simulink model "MPCtest3"  (Simulink 7.9)
settings: Solver=ode45  SolverMode=SingleTasking  StartTime=0  StopTime=100  FixedStep=0.002  RelTol=1e-3  AbsTol=1e-6
libraries: Solver_SF x1
settings Model: Creator=DELL  LastModifiedBy=DELL  ExtModeTrigMode=oneshot  ExtModeArmWhenConnect=off
settings DataIOCC: LimitDataPoints=off  SignalLoggingName=sigsOut
settings OptimizationCC: BlockReduction=off  BooleanDataType=off
settings DebuggingCC: SaveWithParameterizedLinksMsg=none  SignalResolutionControl=TryResolveAllWithWarning  SolverPrmCheckMsg=none  MultiTaskDSMMsg=warning  MultiTaskCondExecSysMsg=none  StrictBusMsg=None
settings HardwareCC: TargetUnknown=on
settings RTWCC: TemplateMakefile=grt_vc.tmf  IncludeERTFirstTime=on
settings GRTTargetCC: TargetFcnLib=ansi_tfl_tmw.mat  CombineOutputUpdateFcns=off  GRTInterface=on

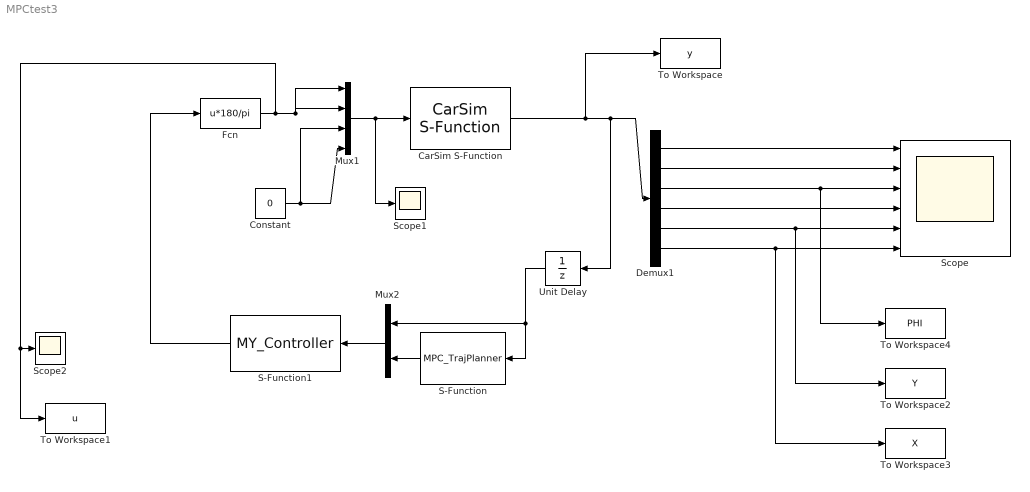
== system MPCtest3 ==
  CarSim S-Function : Solver_SF/CarSim S-Function  Priority=1  VehicleCode=i_i  SIMFILE=simfile
  Constant : Constant  Value=0
  Demux1 : Demux  Outputs=[1 1 1 1 1 1]
  Fcn : Fcn  Expr=u*180/pi
  Mux1 : Mux
  Mux2 : Mux  Inputs=2
  S-Function : S-Function  FunctionName=MPC_TrajPlanner  EnableBusSupport=off
  S-Function1 : S-Function  FunctionName=MY_Controller  EnableBusSupport=off
  Scope : Scope  NumInputPorts=6
      settings: ShowLegends=on  TimeRange=20  YMin=-30~55~-30~-75~-3~25  YMax=30~72.5~30~75~4~225
  Scope1 : Scope
  Scope2 : Scope
      settings: YMin=-0.9  YMax=0.9  SaveName=ScopeData2
  To Workspace : ToWorkspace  VariableName=y  SampleTime=-1  SaveFormat=Timeseries
  To Workspace1 : ToWorkspace  VariableName=u  SampleTime=-1  SaveFormat=Timeseries
  To Workspace2 : ToWorkspace  VariableName=Y  SampleTime=-1  SaveFormat=Timeseries
  To Workspace3 : ToWorkspace  VariableName=X  SampleTime=-1  SaveFormat=Timeseries
  To Workspace4 : ToWorkspace  VariableName=PHI  SampleTime=-1  SaveFormat=Timeseries
  Unit Delay : UnitDelay  SampleTime=-1
  wires:
  CarSim S-Function/1 -> To Workspace/1, Demux1/1, Unit Delay/1
  Unit Delay/1 -> S-Function/1, Mux2/1
  Mux1/1 -> CarSim S-Function/1, Scope1/1
  Fcn/1 -> Mux1/1, Mux1/2, Scope2/1, To Workspace1/1
  Constant/1 -> Mux1/3, Mux1/4
  Mux2/1 -> S-Function1/1
  S-Function/1 -> Mux2/2
  S-Function1/1 -> Fcn/1
  Demux1/1 -> Scope/1
  Demux1/2 -> Scope/2
  Demux1/3 -> Scope/3, To Workspace4/1
  Demux1/4 -> Scope/4
  Demux1/5 -> Scope/5, To Workspace2/1
  Demux1/6 -> Scope/6, To Workspace3/1
